simulink model "rfkjr"  (R2024a)
settings: Solver=FixedStepAuto  StartTime=0.0  StopTime=inf  FixedStep=0.1  RelTol=1e-3
libraries: robotlib x5
settings Model: Creator=ronnie.yalung  LastModifiedBy=JeffZ
settings OptimizationCC: EnhancedBackFolding=on  PassReuseOutputArgsAs=Individual arguments  ZeroExternalMemoryAtStartup=off  ZeroInternalMemoryAtStartup=off  MaxStackSize=64  OptimizeBlockOrder=speed  DifferentSizesBufferReuse=on  OptimizationCustomize=off  EfficientTunableParamExpr=on
settings DebuggingCC: ParameterTunabilityLossMsg=error
settings HardwareCC: ProdBitPerPointer=32  ProdBitPerSizeT=32  ProdBitPerPtrDiffT=32  ProdLargestAtomicFloat=None  ProdIntDivRoundTo=Undefined  ProdEndianess=Unspecified  ProdWordSize=32  ProdHWDeviceType=Generic->Unspecified (assume 32-bit Generic)  UseEmbeddedCoderFeatures=off
settings SFSimCC: MATLABDynamicMemAlloc=off
settings RTWCC: Description=Embedded Coder  SystemTargetFile=ert.tlc  HardwareBoard=Robot Operating System (ROS)  TLCOptions="-aInlineSetEventsForThisBaseRateFcn=TLC_FALSE -aSuppressMultiTaskScheduler=TLC_FALSE  -aRateBasedStepFcn=0"  TemplateMakefile=ert_default_tmf  Toolchain=Catkin  TargetLang=C++
settings CodeAppCC: ForceParamTrailComments=on  IgnoreCustomStorageClasses=off  OperatorAnnotations=on  SimulinkDataObjDesc=on  SFDataObjDesc=on  InsertBlockDesc=on
settings ERTTargetCC: SupportNonInlinedSFcns=on

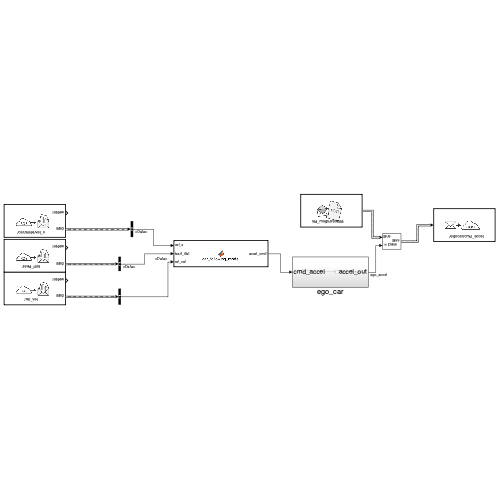
[thumbnail: Simulink's stored preview of the top-level diagram]
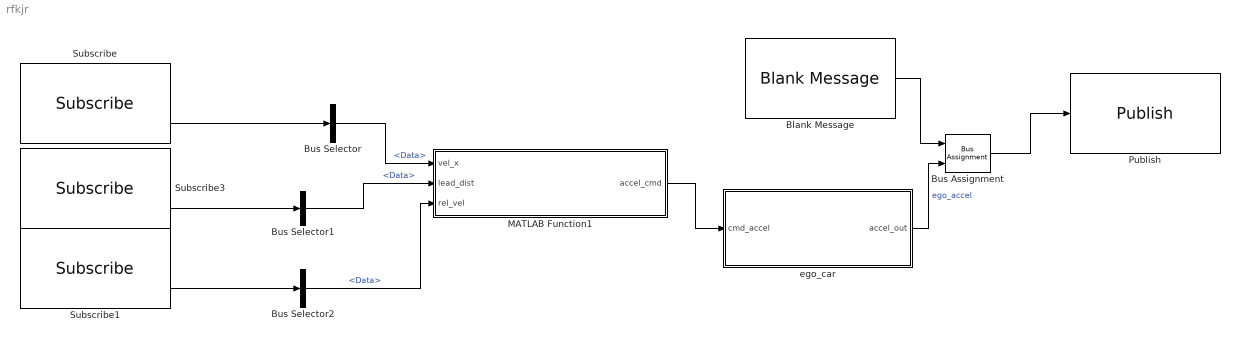
== system rfkjr ==
  Blank Message : robotlib/Blank Message  messageClass=Message  entityType=std_msgs/Float64  messageType=std_msgs/Float64  SampleTime=inf  legacyBusStruct=off
  Bus Assignment : BusAssignment  AssignedSignals=Data
  Bus Selector : BusSelector  OutputSignals=Data
  Bus Selector1 : BusSelector  OutputSignals=Data
  Bus Selector2 : BusSelector  OutputSignals=Data
  MATLAB Function1 : MATLAB Function  TreatAsAtomicUnit=on
  Publish : robotlib/Publish  topicSource=Specify your own  topic=/egocar/cmd_accel  messageType=std_msgs/Float64  legacyBusStruct=off  messageQueueLength=1
  Subscribe : robotlib/Subscribe  topicSource=Specify your own  topic=/car/state/vel_x  messageType=std_msgs/Float64  SampleTime=-1  legacyBusStruct=off  messageQueueLength=1
  Subscribe1 : robotlib/Subscribe  topicSource=Specify your own  topic=/rel_vel  messageType=std_msgs/Float64  SampleTime=-1  legacyBusStruct=off  messageQueueLength=1
  Subscribe3 : robotlib/Subscribe  topicSource=Specify your own  topic=/lead_dist  messageType=std_msgs/Float64  SampleTime=-1  legacyBusStruct=off  messageQueueLength=1
  ego_car : Subsystem
  wires:
  MATLAB Function1/1(accel_cmd) -> ego_car/1(cmd_accel)
  Bus Assignment/1 -> Publish/1
  Blank Message/1 -> Bus Assignment/1
  ego_car/1(accel_out) -> Bus Assignment/2  "ego_accel"
  Subscribe/2 -> Bus Selector/1
  Bus Selector/1 -> MATLAB Function1/1(vel_x)  "<Data>"
  Subscribe3/2 -> Bus Selector1/1
  Bus Selector1/1 -> MATLAB Function1/2(lead_dist)  "<Data>"
  Subscribe1/2 -> Bus Selector2/1
  Bus Selector2/1 -> MATLAB Function1/3(rel_vel)  "<Data>"

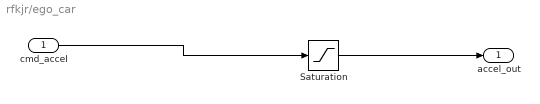
== system rfkjr/ego_car ==
  cmd_accel : Inport
  Saturation : Saturate  UpperLimit=5  LowerLimit=-5
  accel_out : Outport
  wires:
  Saturation/1 -> accel_out/1
  cmd_accel/1 -> Saturation/1

== matlab function rfkjr/MATLAB Function1 ==
  data: accel_cmd output; vel_x input; lead_dist input; rel_vel input
function accel_cmd = car_following_model(vel_x, lead_dist, rel_vel)
    % Eco-Driving Car Following Model with Extended Logic for Large Lead Distance
    % Inputs:
    %   vel_x: Velocity of the ego vehicle (m/s)
    %   lead_dist: Distance to the lead vehicle (m)
    %   rel_vel: Relative velocity between the ego and lead vehicle (lead_vel - ego_vel) (m/s)
    %
    % Output:
    %   accel_cmd: Desired acceleration for the ego vehicle (m/s^2)

    % Parameters for maintaining a safe following distance
    alpha = .5;        % Proportional gain for distance maintenance
    tau = 2.5;          % Desired time gap (seconds)
    
    % Parameters for smooth driving
    beta_acc = 0.05;     % Proportional gain for acceleration smoothness
    beta_dec = 0.25;     % Proportional gain for deceleration smoothness
    max_acc = 1.5;      % Maximum acceleration allowed (m/s^2)
    max_dec = -2.0;     % Maximum deceleration allowed (m/s^2)
    
    % Constant speed parameters
    eco_speed = 20;     % Eco-friendly cruising speed (m/s)
    max_lead_dist = 100; % Maximum distance before ego maintains constant speed (meters)

    % Calculate the desired safe distance using the time gap policy
    desired_space_gap = vel_x * tau;

    % Calculate the error in the current space gap
    gap_error = lead_dist - desired_space_gap;

    % Basic constant time gap control law for maintaining safe distance
    accel_gap_control = alpha * gap_error;

    % Smooth adjustment to avoid abrupt acceleration and braking
    if rel_vel > 0
        % Ego vehicle should accelerate to close the gap
        accel_smooth_control = beta_acc * rel_vel;
    else
        % Ego vehicle should decelerate to maintain gap smoothly
        accel_smooth_control = beta_dec * rel_vel;
    end

    % Desired acceleration is a combination of gap maintenance and smoothness control
    accel_cmd = accel_gap_control + accel_smooth_control;

    % Additional logic for when the lead car is too far away
    if lead_dist > max_lead_dist
        % Maintain a constant speed at the eco-friendly rate
        if vel_x < eco_speed
            % Accelerate to reach eco speed
            accel_cmd = beta_acc * (eco_speed - vel_x);
        elseif vel_x > eco_speed
            % Decelerate to reach eco speed
            accel_cmd = beta_dec * (eco_speed - vel_x);
        else
            % No change in acceleration needed if at desired eco speed
            accel_cmd = 0;
        end
    end

    % Limit acceleration to ensure eco-friendly driving behavior
    accel_cmd = min(max(accel_cmd, max_dec), max_acc);
end
